simulink model "daolibai_zhixian_modbus"  (R2020b)
settings: Solver=ode45  StartTime=0.0  StopTime=100  RelTol=1e-3  EnableMultiTasking=on
settings Model: Creator=passoni  LastModifiedBy=chong
settings DataIOCC: LimitDataPoints=on  SaveFormat=Array  ReturnWorkspaceOutputs=off
settings OptimizationCC: LifeSpan=inf
settings DebuggingCC: SolverPrmCheckMsg=warning  SFUnexpectedBacktrackingDiag=warning  SFNoUnconditionalDefaultTransitionDiag=warning  SFExecutionAtInitializationDiag=none  ArithmeticOperatorsInVariantConditions=warning
settings HardwareCC: ProdBitPerPointer=32  ProdBitPerSizeT=32  ProdBitPerPtrDiffT=32  ProdLargestAtomicFloat=None  ProdIntDivRoundTo=Undefined  ProdEndianess=Unspecified  ProdWordSize=32  ProdHWDeviceType=32-bit Generic
settings ModelReferenceCC: PropagateSignalLabelsOutOfModel=off
settings SFSimCC: SimUseLocalCustomCode=off  CustomCodeUndefinedFunction=UseInterfaceOnly
settings RTWCC: RTWUseLocalCustomCode=off
settings CodeAppCC: StateflowObjectComments=on
settings GRTTargetCC: TargetLangStandard=C89/C90 (ANSI)
settings ConfigComp: CovMetricSettings=dw  CovSaveCumulativeToWorkspaceVar=on  CovSaveSingleToWorkspaceVar=on  CovExternalEMLEnable=off  CovSFcnEnable=off

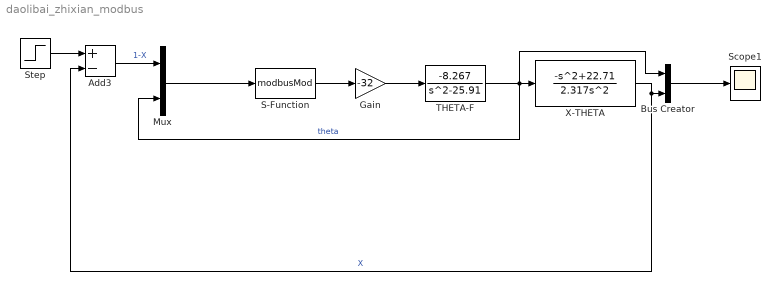
== system daolibai_zhixian_modbus ==
  Add3 : Sum  Inputs=+-
  Bus Creator : BusCreator  Inputs=2
  Gain : Gain  Gain=-32
  Mux : Mux  Inputs=2
  S-Function : S-Function  FunctionName=modbusMod  SFunctionDeploymentMode=off  EnableBusSupport=off
  Scope1 : Scope
  Step : Step  SampleTime=0
  THETA-F : TransferFcn  Numerator=[-8.267]  Denominator=[1 0 -25.91]
  X-THETA : TransferFcn  Numerator=[-1 0 22.71]  Denominator=[2.317 0 0]
  wires:
  Gain/1 -> THETA-F/1
  Bus Creator/1 -> Scope1/1
  Step/1 -> Add3/1
  X-THETA/1 -> Add3/2, Bus Creator/2  "X"
  THETA-F/1 -> Mux/2, X-THETA/1, Bus Creator/1  "theta"
  S-Function/1 -> Gain/1
  Add3/1 -> Mux/1  "1-X"
  Mux/1 -> S-Function/1
